simulink model "o1_ar_filter_optimization_sim"  (R2020b)
settings: Solver=FixedStepDiscrete  StartTime=0.0  StopTime=stopTime  RelTol=1e-3
InitFcn:
  | initCallback
StopFcn:
  | stopCallback
values from neighbouring files (symbols this model uses):
  buf_random_in = rand(1,1)    [modelparameters.m]
  c1_random_in = rand(1,1)    [modelparameters.m]
  c2_random_in = rand(1,1)    [modelparameters.m]
undefined symbols (not defined in the file or in its folder): mp
settings Model: Creator=Ross  LastModifiedBy=conno
settings DataIOCC: ReturnWorkspaceOutputs=off
settings OptimizationCC: BlockReduction=off  ConditionallyExecuteInputs=off  DefaultParameterBehavior=Inlined
settings DebuggingCC: ReadBeforeWriteMsg=DisableAll  WriteAfterWriteMsg=DisableAll  WriteAfterReadMsg=DisableAll  AlgebraicLoopMsg=error  MultiTaskDSMMsg=none  SingleTaskRateTransMsg=error  PregeneratedLibrarySubsystemCodeDiagnostic=none  ArithmeticOperatorsInVariantConditions=warning
settings HardwareCC: ProdBitPerPointer=32  ProdBitPerSizeT=32  ProdBitPerPtrDiffT=32  ProdLargestAtomicFloat=None  ProdIntDivRoundTo=Undefined  ProdEndianess=Unspecified  ProdWordSize=32  ProdHWDeviceType=ASIC/FPGA->ASIC/FPGA  TargetBitPerPointer=64  TargetBitPerSizeT=64  TargetBitPerPtrDiffT=64  TargetLongLongMode=on  TargetIntDivRoundTo=Zero  TargetEndianess=LittleEndian  TargetWordSize=64  TargetHWDeviceType=Custom Processor->MATLAB Host Computer  ProdEqTarget=off
settings ModelReferenceCC: UpdateModelReferenceTargets=IfOutOfDate
settings SFSimCC: SFSimEcho=off  SimUseLocalCustomCode=off  CustomCodeUndefinedFunction=UseInterfaceOnly
settings RTWCC: RTWUseLocalCustomCode=off

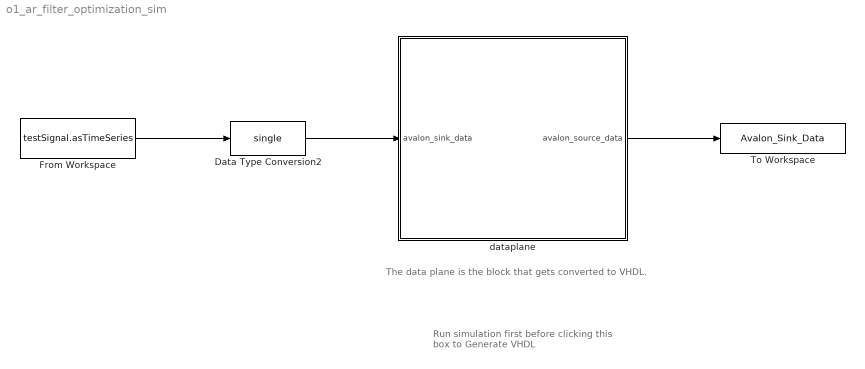
== system o1_ar_filter_optimization_sim ==
  note: The data plane is the block that gets converted to VHDL.
  note: Run simulation first
      | before clicking this box to
      | Generate VHDL
  Data Type Conversion2 : DataTypeConversion  OutDataTypeStr=single  RndMeth=Nearest
  From Workspace : FromWorkspace  VariableName=testSignal.asTimeSeries  SampleTime=mp.Ts
  To Workspace : ToWorkspace  VariableName=Avalon_Sink_Data  SampleTime=-1
  dataplane : Subsystem  TreatAsAtomicUnit=on
  wires:
  From Workspace/1 -> Data Type Conversion2/1
  Data Type Conversion2/1 -> dataplane/1(avalon_sink_data)
  dataplane/1(avalon_source_data) -> To Workspace/1

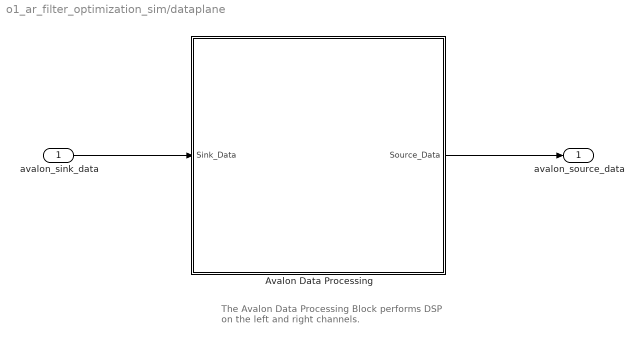
== system o1_ar_filter_optimization_sim/dataplane ==
  note: The Avalon Data Processing Block
      | performs DSP on the left and right channels.
  avalon_sink_data : Inport
  Avalon Data Processing : Subsystem  TreatAsAtomicUnit=on
  avalon_source_data : Outport  VectorParamsAs1DForOutWhenUnconnected=off
  wires:
  Avalon Data Processing/1(Source_Data) -> avalon_source_data/1
  avalon_sink_data/1 -> Avalon Data Processing/1(Sink_Data)

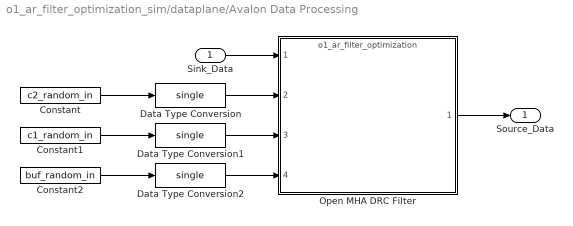
== system o1_ar_filter_optimization_sim/dataplane/Avalon Data Processing ==
  Sink_Data : Inport
  Constant : Constant  Value=c2_random_in  SampleTime=-1
  Constant1 : Constant  Value=c1_random_in  SampleTime=-1
  Constant2 : Constant  Value=buf_random_in  SampleTime=-1
  Data Type Conversion : DataTypeConversion  OutDataTypeStr=single  RndMeth=Nearest
  Data Type Conversion1 : DataTypeConversion  OutDataTypeStr=single  RndMeth=Nearest
  Data Type Conversion2 : DataTypeConversion  OutDataTypeStr=single  RndMeth=Nearest
  Open MHA DRC Filter : ModelReference  ModelNameDialog=o1_ar_filter_optimization.slx  SimulationMode=Normal  ModelReferenceVersion=1.139
  Source_Data : Outport  InitialOutput=0  VectorParamsAs1DForOutWhenUnconnected=off
  wires:
  Sink_Data/1 -> Open MHA DRC Filter/1
  Data Type Conversion2/1 -> Open MHA DRC Filter/4
  Data Type Conversion1/1 -> Open MHA DRC Filter/3
  Data Type Conversion/1 -> Open MHA DRC Filter/2
  Constant/1 -> Data Type Conversion/1
  Constant1/1 -> Data Type Conversion1/1
  Constant2/1 -> Data Type Conversion2/1
  Open MHA DRC Filter/1 -> Source_Data/1
